simulink model "remap_axis"  (R2023b)
settings: Solver=VariableStepAuto  StartTime=0.0  StopTime=671  RelTol=1e-3
libraries: dspstat3 x6, matrix_library x1, vrlib x1
settings Model: Creator=TAK  LastModifiedBy=TAK
settings DataIOCC: ExternalInput=Sheet1.getElement('accel_x'),Sheet1.getElement('accel_y'),Sheet1.getElement('accel_z'),Sheet1.getElement('gyro_x'),Sheet1.getElement('gyro_y'),Sheet1.getElement('gyro_z'),Sheet1.getElement('hv_on'),Sheet1.getElement('rtd')  LoadExternalInput=on

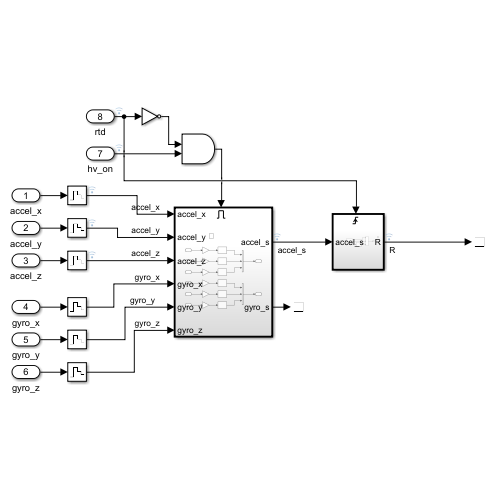
[thumbnail: Simulink's stored preview of the top-level diagram]
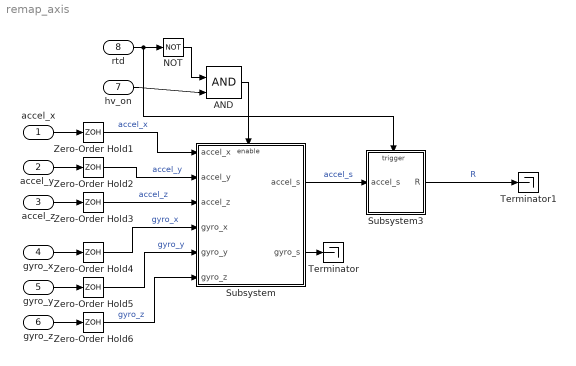
== system remap_axis ==
  accel_x : Inport  PortDimensions=1
  accel_y : Inport  Port=2  PortDimensions=1
  accel_z : Inport  Port=3  PortDimensions=1
  gyro_x : Inport  Port=4  PortDimensions=1
  gyro_y : Inport  Port=5  PortDimensions=1
  gyro_z : Inport  Port=6  PortDimensions=1
  hv_on : Inport  Port=7
  rtd : Inport  Port=8
  AND : Logic  IconShape=distinctive  AllPortsSameDT=off  OutDataTypeStr=boolean
  NOT : Logic  Operator=NOT  IconShape=distinctive  AllPortsSameDT=off  OutDataTypeStr=boolean
  Subsystem : Subsystem
  Subsystem3 : Subsystem
  Terminator : Terminator
  Terminator1 : Terminator
  Zero-Order Hold{1..6} (6 alike) : ZeroOrderHold  SampleTime=.02
  wires:
  accel_x/1 -> Zero-Order Hold1/1
  accel_y/1 -> Zero-Order Hold2/1
  accel_z/1 -> Zero-Order Hold3/1
  gyro_x/1 -> Zero-Order Hold4/1
  gyro_y/1 -> Zero-Order Hold5/1
  gyro_z/1 -> Zero-Order Hold6/1
  Subsystem/2(gyro_s) -> Terminator/1
  Subsystem/1(accel_s) -> Subsystem3/1(accel_s)  "accel_s"
  Subsystem3/1(R) -> Terminator1/1  "R"
  AND/1 -> Subsystem/Enable
  rtd/1 -> Subsystem3/Trigger, NOT/1
  NOT/1 -> AND/1
  hv_on/1 -> AND/2
  Zero-Order Hold1/1 -> Subsystem/1(accel_x)  "accel_x"
  Zero-Order Hold2/1 -> Subsystem/2(accel_y)  "accel_y"
  Zero-Order Hold3/1 -> Subsystem/3(accel_z)  "accel_z"
  Zero-Order Hold4/1 -> Subsystem/4(gyro_x)  "gyro_x"
  Zero-Order Hold5/1 -> Subsystem/5(gyro_y)  "gyro_y"
  Zero-Order Hold6/1 -> Subsystem/6(gyro_z)  "gyro_z"

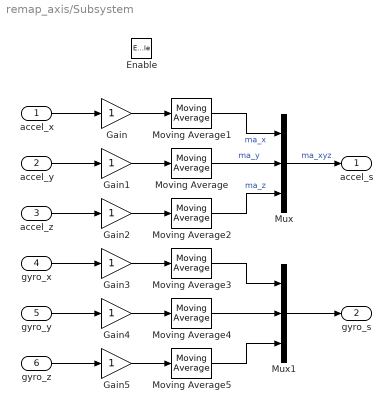
== system remap_axis/Subsystem ==
  accel_x : Inport
  accel_y : Inport  Port=2
  accel_z : Inport  Port=3
  gyro_x : Inport  Port=4
  gyro_y : Inport  Port=5
  gyro_z : Inport  Port=6
  Enable : EnablePort
  Gain{,1..5} (6 alike) : Gain
  Moving Average : dspstat3/Moving Average  Method=Sliding window  ForgettingFactorPort=off  SpecifyWindowLength=off  WindowLength=4  OverlapLength=3  AllowArbitraryInputLength=off  ForgettingFactor=0.9  SimulateUsing=Code generation
  Moving Average1 : dspstat3/Moving Average  Method=Sliding window  ForgettingFactorPort=off  SpecifyWindowLength=off  WindowLength=4  OverlapLength=3  AllowArbitraryInputLength=off  ForgettingFactor=0.9  SimulateUsing=Code generation
  Moving Average2 : dspstat3/Moving Average  Method=Sliding window  ForgettingFactorPort=off  SpecifyWindowLength=off  WindowLength=4  OverlapLength=3  AllowArbitraryInputLength=off  ForgettingFactor=0.9  SimulateUsing=Code generation
  Moving Average3 : dspstat3/Moving Average  Method=Sliding window  ForgettingFactorPort=off  SpecifyWindowLength=on  WindowLength=4  OverlapLength=3  AllowArbitraryInputLength=off  ForgettingFactor=0.9  SimulateUsing=Code generation
  Moving Average4 : dspstat3/Moving Average  Method=Sliding window  ForgettingFactorPort=off  SpecifyWindowLength=on  WindowLength=4  OverlapLength=3  AllowArbitraryInputLength=off  ForgettingFactor=0.9  SimulateUsing=Code generation
  Moving Average5 : dspstat3/Moving Average  Method=Sliding window  ForgettingFactorPort=off  SpecifyWindowLength=on  WindowLength=4  OverlapLength=3  AllowArbitraryInputLength=off  ForgettingFactor=0.9  SimulateUsing=Code generation
  Mux : Mux  Inputs=3
  Mux1 : Mux  Inputs=3
  accel_s : Outport
  gyro_s : Outport  Port=2
  wires:
  accel_y/1 -> Gain1/1
  Mux/1 -> accel_s/1  "ma_xyz"
  Gain2/1 -> Moving Average2/1
  Moving Average4/1 -> Mux1/2
  gyro_y/1 -> Gain4/1
  Gain4/1 -> Moving Average4/1
  Gain3/1 -> Moving Average3/1
  gyro_z/1 -> Gain5/1
  Moving Average/1 -> Mux/2  "ma_y"
  Mux1/1 -> gyro_s/1
  Moving Average2/1 -> Mux/3  "ma_z"
  accel_z/1 -> Gain2/1
  accel_x/1 -> Gain/1
  Moving Average1/1 -> Mux/1  "ma_x"
  Gain1/1 -> Moving Average/1
  Moving Average5/1 -> Mux1/3
  Gain5/1 -> Moving Average5/1
  Moving Average3/1 -> Mux1/1
  Gain/1 -> Moving Average1/1
  gyro_x/1 -> Gain3/1

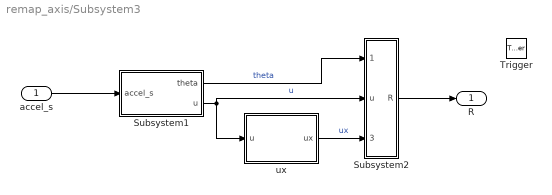
== system remap_axis/Subsystem3 ==
  accel_s : Inport
  Trigger : TriggerPort  VariantControl=(inherit)  PortDimensions=1
  Subsystem1 : Subsystem
  Subsystem2 : Subsystem
  ux : MATLAB Function  TreatAsAtomicUnit=on
  R : Outport
  wires:
  ux/1(ux) -> Subsystem2/3(ux)  "ux"
  Subsystem1/2(u) -> ux/1(u), Subsystem2/2(u)  "u"
  Subsystem1/1(theta) -> Subsystem2/1(theta)  "theta"
  Subsystem2/1(R) -> R/1
  accel_s/1 -> Subsystem1/1(accel_s)

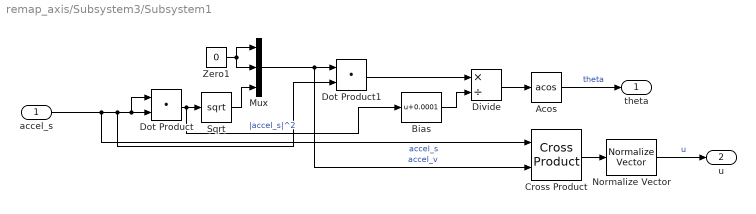
== system remap_axis/Subsystem3/Subsystem1 ==
  accel_s : Inport  PortDimensions=[3 1]
  Acos : Trigonometry  Operator=acos
  Bias : Bias  Bias=0.0001  SaturateOnIntegerOverflow=off
  Cross Product : matrix_library/Cross Product
  Divide : Product  Inputs=*/
  Dot Product : DotProduct  OutDataTypeStr=Inherit: Inherit via internal rule
  Dot Product1 : DotProduct  OutDataTypeStr=Inherit: Inherit via internal rule
  Mux : Mux  Inputs=3
  Normalize Vector : vrlib/Utilities/Normalize Vector  maxzero=0
  Sqrt : Sqrt
  Zero1 : Constant  Value=0  OutDataTypeStr=Inherit: Inherit via back propagation
  theta : Outport
  u : Outport  Port=2
  wires:
  accel_s/1 -> Cross Product/1, Dot Product1/2, Dot Product/1, Dot Product/2  "accel_s"
  Cross Product/1 -> Normalize Vector/1
  Dot Product1/1 -> Divide/1
  Normalize Vector/1 -> u/1  "u"
  Dot Product/1 -> Bias/1, Sqrt/1  "|accel_s|^2"
  Sqrt/1 -> Mux/3
  Mux/1 -> Cross Product/2, Dot Product1/1  "accel_v"
  Zero1/1 -> Mux/1, Mux/2
  Divide/1 -> Acos/1
  Acos/1 -> theta/1  "theta"
  Bias/1 -> Divide/2

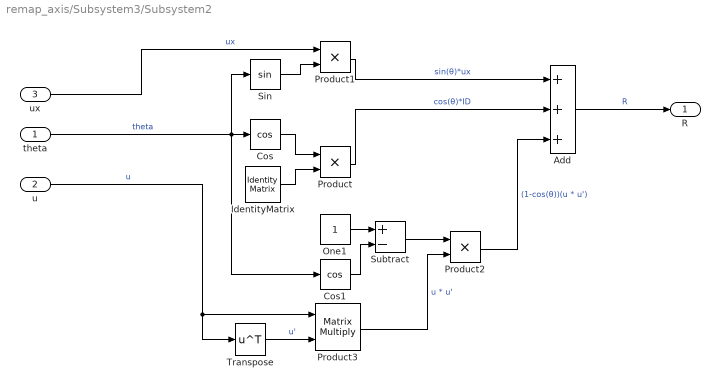
== system remap_axis/Subsystem3/Subsystem2 ==
  theta : Inport
  u : Inport  Port=2
  ux : Inport  Port=3
  Add : Sum  Inputs=+++
  Cos : Trigonometry  Operator=cos
  Cos1 : Trigonometry  Operator=cos
  IdentityMatrix : IdentityMatrix  OutputDimensions=3  SampleTime=-1
  One1 : Constant  OutDataTypeStr=Inherit: Inherit via back propagation
  Product : Product
  Product1 : Product
  Product2 : Product
  Product3 : Product  Multiplication=Matrix(*)
  Sin : Trigonometry
  Subtract : Sum  Inputs=+-
  Transpose : Math  Operator=transpose
  R : Outport
  wires:
  theta/1 -> Cos1/1, Sin/1, Cos/1  "theta"
  Product/1 -> Add/2  "cos(θ)*ID"
  Cos1/1 -> Subtract/2
  Cos/1 -> Product/1
  Subtract/1 -> Product2/1
  ux/1 -> Product1/1  "ux"
  One1/1 -> Subtract/1
  IdentityMatrix/1 -> Product/2
  u/1 -> Product3/1, Transpose/1  "u"
  Sin/1 -> Product1/2
  Product1/1 -> Add/1  "sin(θ)*ux"
  Add/1 -> R/1  "R"
  Transpose/1 -> Product3/2  "u'"
  Product2/1 -> Add/3  "(1-cos(θ))(u * u')"
  Product3/1 -> Product2/2  "u * u'"

== matlab function remap_axis/Subsystem3/ux ==
  data: u input size=[3 1]; ux output
function ux = fcn(u)

ux = [0 -u(3) u(2); u(3) 0 -u(1); -u(2) u(1) 0];
